simulink model "test_loop_interno1"  (R2020a)
settings: Solver=ode4  StartTime=0.0  StopTime=10  FixedStep=0.00001  RelTol=1e-3
undefined symbols (not defined in the file or in its folder): denC0d, G, numC0d, pi_pos
settings Model: Creator=edoar  LastModifiedBy=edoar

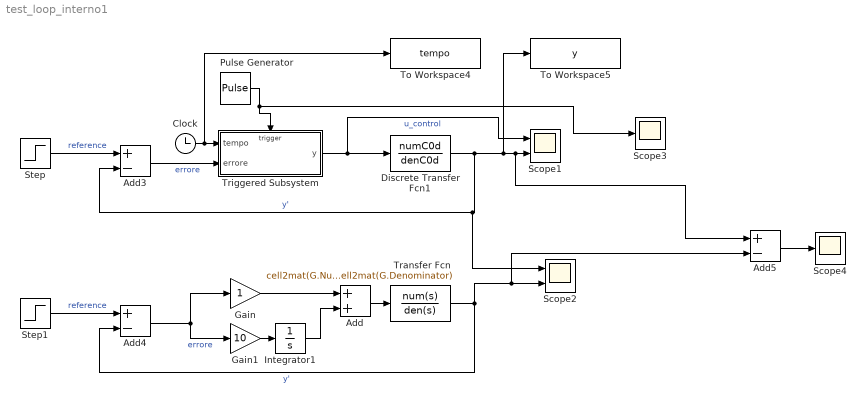
== system test_loop_interno1 ==
  Add : Sum
  Add3 : Sum  Inputs=+-
  Add4 : Sum  Inputs=+-
  Add5 : Sum  Inputs=+-
  Clock : Clock
  Discrete Transfer Fcn1 : DiscreteTransferFcn  Numerator=numC0d  Denominator=denC0d
  Gain : Gain
  Gain1 : Gain  Gain=10
  Integrator1 : Integrator
  Pulse Generator : DiscretePulseGenerator  PulseType=Time based  Period=0.001  PulseWidth=50
  Scope1 : Scope  NumInputPorts=2
  Scope2 : Scope  NumInputPorts=2
  Scope3 : Scope
  Scope4 : Scope
  Step : Step  Time=0  SampleTime=0
  Step1 : Step  Time=0  SampleTime=0
  To Workspace4 : ToWorkspace  VariableName=tempo  SaveFormat=Timeseries  SampleTime=-1
  To Workspace5 : ToWorkspace  VariableName=y  SaveFormat=Timeseries  SampleTime=-1
  Transfer Fcn : TransferFcn  Numerator=cell2mat(G.Numerator)  Denominator=cell2mat(G.Denominator)
  Triggered Subsystem : Subsystem  TreatAsAtomicUnit=on
  wires:
  Pulse Generator/1 -> Triggered Subsystem/Trigger, Scope3/1
  Step/1 -> Add3/1  "reference"
  Triggered Subsystem/1(y) -> Scope1/1, Discrete Transfer Fcn1/1  "u_control"
  Discrete Transfer Fcn1/1 -> To Workspace5/1, Add5/1, Scope1/2, Scope2/1, Add3/2  "y'"
  Add3/1 -> Triggered Subsystem/2(errore)  "errore"
  Clock/1 -> To Workspace4/1, Triggered Subsystem/1(tempo)
  Transfer Fcn/1 -> Add5/2, Scope2/2, Add4/2  "y'"
  Step1/1 -> Add4/1  "reference"
  Gain/1 -> Add/1
  Gain1/1 -> Integrator1/1
  Integrator1/1 -> Add/2
  Add4/1 -> Gain1/1, Gain/1  "errore"
  Add/1 -> Transfer Fcn/1
  Add5/1 -> Scope4/1

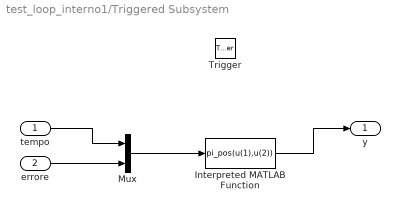
== system test_loop_interno1/Triggered Subsystem ==
  tempo : Inport
  errore : Inport  Port=2
  Trigger : TriggerPort  VariantControl=Variant
  Interpreted MATLAB Function : MATLABFcn  MATLABFcn=pi_pos(u(1),u(2))
  Mux : Mux  Inputs=2
  y : Outport
  wires:
  tempo/1 -> Mux/1
  errore/1 -> Mux/2
  Mux/1 -> Interpreted MATLAB Function/1
  Interpreted MATLAB Function/1 -> y/1
